simulink library "Gear_Selection_Library"  (R2025b)
settings: Solver=VariableStepAuto  StartTime=0.0  StopTime=10.0  RelTol=1e-3

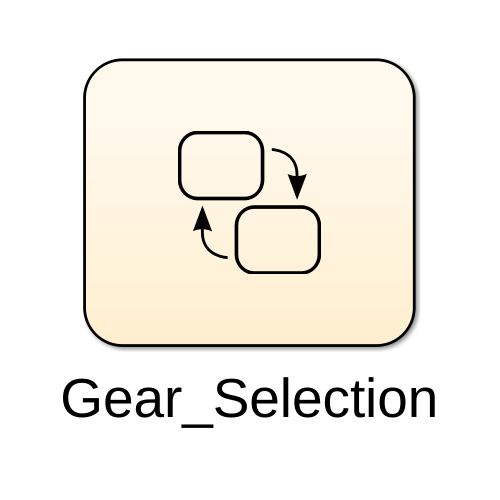
[thumbnail: Simulink's stored preview of the top-level diagram]
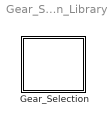
== system Gear_Selection_Library ==
  Gear_Selection : Stateflow chart  TreatAsAtomicUnit=on

== stateflow chart Gear_Selection_Library/Gear_Selection ==
  state Drive
    entry:
    Current_Gear = D;
    state FirstSpeed
      entry:
      Current_Gear = 1;
      UpShift = 0;
      DownShift = 0;
      during:
      Shift_Solenoid_A=0;
      Shift_Solenoid_B=0;
      Shift_Solenoid_C=1;
      Shift_Solenoid_D=1;
      Shift_Solenoid_E=0;
      exit:
    state SecondSpeed
      entry:
      Current_Gear = 2;
      UpShift = 0;
      DownShift = 0;
      during:
      Shift_Solenoid_A=0;
      Shift_Solenoid_B=0;
      Shift_Solenoid_C=1;
      Shift_Solenoid_D=0;
      Shift_Solenoid_E=1;
      exit:
    state ThirdSpeed
      entry:
      Current_Gear = 3;
      UpShift = 0;
      DownShift = 0;
      during:
      Shift_Solenoid_A=1;
      Shift_Solenoid_B=0;
      Shift_Solenoid_C=1;
      Shift_Solenoid_D=0;
      Shift_Solenoid_E=0;
      exit:
    state FourthSpeed
      entry:
      Current_Gear = 4;
      UpShift = 0;
      DownShift = 0;
      during:
      Shift_Solenoid_A=0;
      Shift_Solenoid_B=1;
      Shift_Solenoid_C=1;
      Shift_Solenoid_D=0;
      Shift_Solenoid_E=0;
      exit:
    state FifthSpeed
      entry:
      Current_Gear = 5;
      UpShift = 0;
      DownShift = 0;
      during:
      Shift_Solenoid_A=1;
      Shift_Solenoid_B=1;
      Shift_Solenoid_C=0;
      Shift_Solenoid_D=0;
      Shift_Solenoid_E=0;
      exit:
    state SixthSpeed
      entry:
      Current_Gear = 6;
      UpShift = 0;
      DownShift = 0;
      during:
      Shift_Solenoid_A=0;
      Shift_Solenoid_B=1;
      Shift_Solenoid_C=0;
      Shift_Solenoid_D=0;
      Shift_Solenoid_E=1;
      exit:
    (default) -> FirstSpeed
    FirstSpeed -> SecondSpeed : [UpShift == 1]
    SecondSpeed -> FirstSpeed [order 1] : [DownShift == 1]
    SecondSpeed -> ThirdSpeed [order 2] : [UpShift == 1]
    ThirdSpeed -> SecondSpeed [order 1] : [DownShift == 1]
    ThirdSpeed -> FourthSpeed [order 2] : [UpShift == 1]
    FourthSpeed -> ThirdSpeed [order 1] : [DownShift == 1]
    FourthSpeed -> FifthSpeed [order 2] : [UpShift == 1]
    FifthSpeed -> FourthSpeed [order 1] : [DownShift == 1]
    FifthSpeed -> SixthSpeed [order 2] : [UpShift == 1]
    SixthSpeed -> FifthSpeed : [DownShift == 1]
  state Neutral
    entry:
    Current_Gear = N;
    during:
    Shift_Solenoid_A=0;
    Shift_Solenoid_B=0;
    Shift_Solenoid_C=0;
    Shift_Solenoid_D=0;
    Shift_Solenoid_E=0;
  state Parking
    entry:
    Current_Gear = P;
    Shift_Solenoid_A=0;
    Shift_Solenoid_B=0;
    Shift_Solenoid_C=0;
    Shift_Solenoid_D=0;
    Shift_Solenoid_E=0;
    exit:
  state Reverse
    entry:
    Current_Gear = R;
    during:
    Shift_Solenoid_A=1;
    Shift_Solenoid_B=0;
    Shift_Solenoid_C=0;
    Shift_Solenoid_D=1;
    Shift_Solenoid_E=0;
  (default) -> Parking
  Reverse -> Neutral [order 2] : [Gear_Lever_Position == 2 && Brake_Pedal_Switch == 1 && Vehicle_Speed_Reference < 3 ]
  Neutral -> Drive [order 2] : [Gear_Lever_Position == 3 && Brake_Pedal_Switch == 1 && Vehicle_Speed_Reference < 0 ]
  Parking -> Reverse : [Gear_Lever_Position == 1 && Brake_Pedal_Switch == 1 && Vehicle_Speed_Reference < 3 ]
  Neutral -> Reverse [order 1] : [Gear_Lever_Position == 1 && Brake_Pedal_Switch == 1 && Vehicle_Speed_Reference == 0 ]
  Reverse -> Parking [order 1] : [Gear_Lever_Position == 0 && Brake_Pedal_Switch == 1 && Vehicle_Speed_Reference == 0 ]
  Drive -> Neutral : [Gear_Lever_Position == 2 ]
